simulink model "Nonlinear_Rocket_Model"  (R2019a)
settings: Solver=VariableStepAuto  StartTime=0.0  StopTime=75  RelTol=1e-3
libraries: simulink_extras x2, simulink x1
settings Model: Creator=abhi  LastModifiedBy=abhi

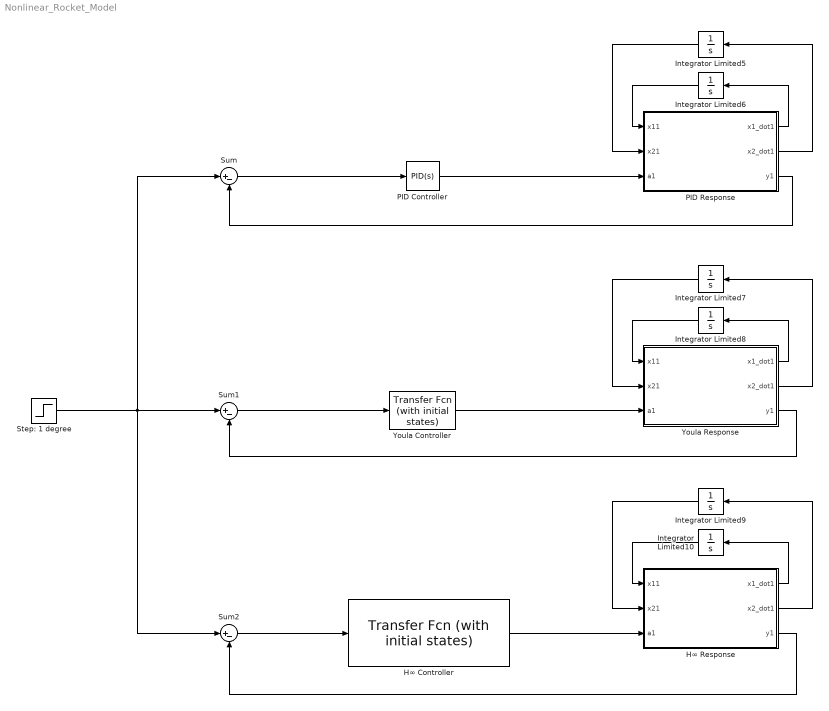
== system Nonlinear_Rocket_Model ==
  H∞ Controller : simulink_extras/Additional Linear/Transfer Fcn (with initial states)  N=[7581 6020 817.6 30.76]  D=[1 155.5 980.7 19.57 0.09775]  X0=0
  H∞ Response : MATLAB Function  TreatAsAtomicUnit=on
  Integrator Limited{5..10} (6 alike) : Integrator  UpperSaturationLimit=1  LowerSaturationLimit=0  IgnoreLimit=on
  "PID Controller " : simulink/Continuous/PID Controller  Controller=PID  Form=Ideal  TimeDomain=Continuous-time  SampleTime=-1  IntegratorMethod=Forward Euler  FilterMethod=Forward Euler  ControllerParametersSource=internal  P=0.825493884458449  I=0.0468147782797737  D=5.24517904929436  UseFilter=on  N=5.45397025421619  TunerSelectOption=Transfer Function Based (PID Tuner App)  InitialConditionSource=internal  InitialConditionForIntegrator=0  InitialConditionForFilter=0  DifferentiatorICPrevScaledInput=0  ExternalReset=none  TrackingMode=off  Kt=1  LimitOutput=off  UpperSaturationLimit=inf  LowerSaturationLimit=-inf  LinearizeAsGain=on  AntiWindupMode=none  Kb=1  POutMin=[]  POutMax=[]  IOutMin=[]  IOutMax=[]  DOutMin=[]  DOutMax=[]  NOutMin=[]  NOutMax=[]  SumOutMin=[]  SumOutMax=[]  SaturationOutMin=[]  SaturationOutMax=[]  PParamMin=[]  PParamMax=[]  IParamMin=[]  IParamMax=[]  DParamMin=[]  DParamMax=[]  NParamMin=[]  NParamMax=[]  KbParamMin=[]  KbParamMax=[]  KtParamMin=[]  KtParamMax=[]  KbOutMin=[]  KbOutMax=[]  KtOutMin=[]  KtOutMax=[]  IntegratorOutMin=[]  IntegratorOutMax=[]  FilterOutMin=[]  FilterOutMax=[]  SumI1OutMin=[]  SumI1OutMax=[]  SumI2OutMin=[]  SumI2OutMax=[]  SumI3OutMin=[]  SumI3OutMax=[]  SumI4OutMin=[]  SumI4OutMax=[]  SumDOutMin=[]  SumDOutMax=[]  DifferentiatorOutMin=[]  DifferentiatorOutMax=[]  FilterDiffOutCoefMin=[]  FilterDiffOutCoefMax=[]  ReciprocalOutMin=[]  ReciprocalOutMax=[]  SumDenOutMin=[]  SumDenOutMax=[]  SumNumOutMin=[]  SumNumOutMax=[]  DivideOutMin=[]  DivideOutMax=[]  IntegratorContinuousStateAttributes=''  IntegratorStateMustResolveToSignalObject=off  IntegratorRTWStateStorageClass=Auto  FilterContinuousStateAttributes=''  FilterStateMustResolveToSignalObject=off  FilterRTWStateStorageClass=Auto  ParallelPVariant=Passthrough  IdealPVariant=InternalParameters  IVariant=InternalParameters  DVariant=InternalParameters  IntegratorVariant=Continuous  SatVariant=Disabled  AWVariant=Passthrough  PCopyVariant=Disabled  TRVariant=Disabled  FdbkBlocksVariant=Forward  IdealPFdbkVariant=Disabled  SatFdbkVariant=Disabled  DerivativeFilterVariant=ContFilter  NVariant=InternalParameters  NCopyVariant=Disabled  FilterICVariant=InternalICsFilter  IntegratorICVariant=InternalICs  ExternalResetVariant=Disabled  TRSumVariant=Passthrough  SumFdbkVariant=Disabled  SumVariant=Sum_PID
  PID Response : MATLAB Function  TreatAsAtomicUnit=on
  Step: 1 degree : Step  Time=10  After=0.017452
  Sum : Sum  Inputs=|+-
  Sum1 : Sum  Inputs=|+-
  Sum2 : Sum  Inputs=|+-
  Youla Controller : simulink_extras/Additional Linear/Transfer Fcn (with initial states)  N=[48.64 27.3]  D="[1  9.702]"  X0=0
  Youla Response : MATLAB Function  TreatAsAtomicUnit=on
  wires:
  PID Response/3(y1) -> Sum/2
  Sum/1 -> "PID Controller "/1
  Sum1/1 -> Youla Controller/1
  Sum2/1 -> H∞ Controller/1
  Step: 1 degree/1 -> Sum/1, Sum2/1, Sum1/1
  PID Response/1(x1_dot1) -> Integrator Limited6/1
  PID Response/2(x2_dot1) -> Integrator Limited5/1
  Integrator Limited5/1 -> PID Response/2(x21)
  Integrator Limited6/1 -> PID Response/1(x11)
  Integrator Limited8/1 -> Youla Response/1(x11)
  Integrator Limited7/1 -> Youla Response/2(x21)
  Youla Response/2(x2_dot1) -> Integrator Limited7/1
  Youla Response/1(x1_dot1) -> Integrator Limited8/1
  "PID Controller "/1 -> PID Response/3(a1)
  H∞ Response/1(x1_dot1) -> Integrator Limited10/1
  H∞ Response/2(x2_dot1) -> Integrator Limited9/1
  Integrator Limited9/1 -> H∞ Response/2(x21)
  Integrator Limited10/1 -> H∞ Response/1(x11)
  Youla Controller/1 -> Youla Response/3(a1)
  H∞ Controller/1 -> H∞ Response/3(a1)
  Youla Response/3(y1) -> Sum1/2
  H∞ Response/3(y1) -> Sum2/2

== matlab function Nonlinear_Rocket_Model/PID Response ==
  data: x1_dot1 output; x11 input; x21 input; x2_dot1 output; a1 input; y1 output
function [x1_dot1, x2_dot1, y1] = fcn(x11, x21, a1)
c1 = 0.1234648871;
c2 = 0.224931119135972;
x1_dot1 = x21;
x2_dot1 = -c1*(sin(x11))^2 + c2*a1; 
y1 = x11;

== matlab function Nonlinear_Rocket_Model/Youla Response ==
  data: x1_dot1 output; x11 input; x21 input; x2_dot1 output; a1 input; y1 output
function [x1_dot1, x2_dot1, y1] = fcn(x11, x21, a1)
c1 = 0.1234648871;
c2 = 0.224931119135972;
x1_dot1 = x21;
x2_dot1 = -c1*(sin(x11))^2 + c2*a1;  
y1 = x11;

== matlab function Nonlinear_Rocket_Model/H∞ Response ==
  data: x1_dot1 output; x11 input; x21 input; x2_dot1 output; a1 input; y1 output
function [x1_dot1, x2_dot1, y1] = fcn(x11, x21, a1)
c1 = 0.1234648871;
c2 = 0.224931119135972;
x1_dot1 = x21;
x2_dot1 = -c1*(sin(x11))^2 + c2*a1;
y1 = x11;
